simulink model "SOC_Estimation"  (R2019b)
settings: configuration reference "BMS_Sw_CodeGenConfig" (kept outside this file)
undefined symbols (not defined in the file): Battery, BMS_State_Enum, DiscIntNeverNeededParam, Ns_Module, NumModules, SOCInit, Ts
libraries: sharedTrackingLibrary x2, simulink x1
settings Model: DataDictionary=DD_SOC_Estimation.sldd  EnableAccessToBaseWorkspace=off  ExtModeTrigDuration=5  Creator=cpatel  LastModifiedBy=cpatel
settings ConfigSetRef: SourceName=BMS_Sw_CodeGenConfig

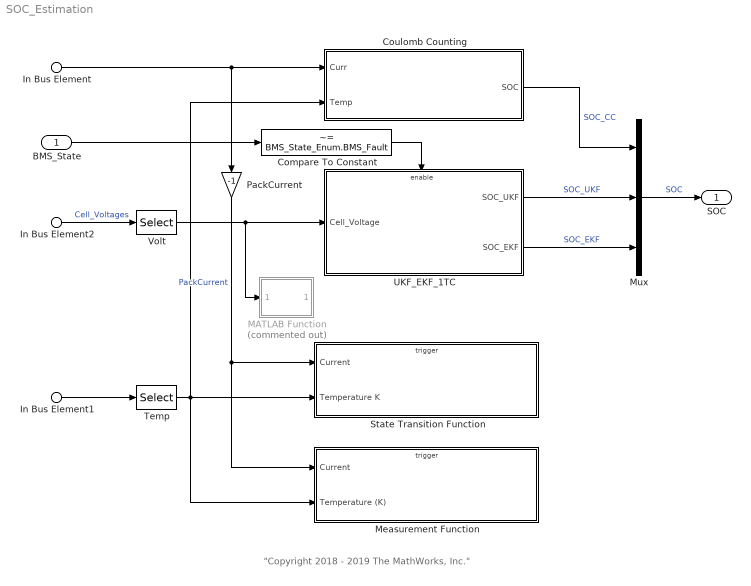
== system SOC_Estimation ==
  note: "Copyright 2018 - 2019 The MathWorks, Inc."
  BMS_State : Inport  OutDataTypeStr=Enum: BMS_State_Enum
  In Bus Element2 : Inport  Port=2  PortName=BMS_Input  Element=Cell_Voltages
  In Bus Element : Inport  Port=2  PortName=BMS_Input  Element=Pack_Current
  In Bus Element1 : Inport  Port=2  PortName=BMS_Input  Element=Cell_Temperatures
  Compare To Constant : simulink/Logic and Bit Operations/Compare To Constant  relop=~=  const=BMS_State_Enum.BMS_Fault  OutDataTypeStr=boolean
  Coulomb Counting : Subsystem  VariantControl=SocAlgo==1
  MATLAB Function : MATLAB Function  Commented=on  TreatAsAtomicUnit=on
  Measurement Function : Subsystem  TreatAsAtomicUnit=on
  Mux : Mux  Inputs=3
  PackCurrent : Gain  Gain=-1
  State Transition Function : Subsystem  TreatAsAtomicUnit=on
  Temp : Selector  InputPortWidth=Ns_Module*NumModules  IndexOptions=Index vector (dialog)  Indices=1  OutputSizes=1
  UKF_EKF_1TC : Subsystem  VariantControl=CellType==1
  Volt : Selector  InputPortWidth=Ns_Module*NumModules  IndexOptions=Index vector (dialog)  Indices=1  OutputSizes=1
  SOC : Outport  OutDataTypeStr=single  SampleTime=[0.10000000000000001,0]  VectorParamsAs1DForOutWhenUnconnected=off
  wires:
  In Bus Element2/1 -> Volt/1  "Cell_Voltages"
  In Bus Element1/1 -> Temp/1
  Mux/1 -> SOC/1  "SOC"
  Coulomb Counting/1(SOC) -> Mux/1  "SOC_CC"
  In Bus Element/1 -> PackCurrent/1, Coulomb Counting/1(Curr)
  UKF_EKF_1TC/1(SOC_UKF) -> Mux/2  "SOC_UKF"
  UKF_EKF_1TC/2(SOC_EKF) -> Mux/3  "SOC_EKF"
  BMS_State/1 -> Compare To Constant/1
  Compare To Constant/1 -> UKF_EKF_1TC/Enable
  PackCurrent/1 -> State Transition Function/1(Current), Measurement Function/1(Current)  "PackCurrent"
  Temp/1 -> State Transition Function/2(Temperature K), Measurement Function/2(Temperature (K)), Coulomb Counting/2(Temp)
  Volt/1 -> UKF_EKF_1TC/1(Cell_Voltage), MATLAB Function/1(meas)

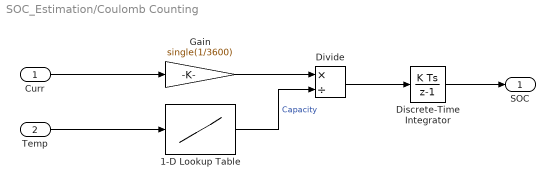
== system SOC_Estimation/Coulomb Counting ==
  Curr : Inport
  Temp : Inport  Port=2
  1-D Lookup Table : Lookup_n-D  NumberOfTableDimensions=1  BreakpointsForDimension1=single(Battery(1).Temperature_LUT)  Table=single(Battery(1).Capacity_LUT)  InternalRulePriority=Speed  RndMeth=Simplest  InputSameDT=on
  Discrete-Time Integrator : DiscreteIntegrator  InitialCondition=single(SOCInit+0.05)  SampleTime=-1  LimitOutput=on  UpperSaturationLimit=1  LowerSaturationLimit=0  ICPrevOutput=DiscIntNeverNeededParam  ICPrevScaledInput=DiscIntNeverNeededParam
  Divide : Product  Inputs=*/
  Gain : Gain  Gain=single(1/3600)
  SOC : Outport  VectorParamsAs1DForOutWhenUnconnected=off
  wires:
  Discrete-Time Integrator/1 -> SOC/1
  Curr/1 -> Gain/1
  Gain/1 -> Divide/1
  Divide/1 -> Discrete-Time Integrator/1
  1-D Lookup Table/1 -> Divide/2  "Capacity"
  Temp/1 -> 1-D Lookup Table/1

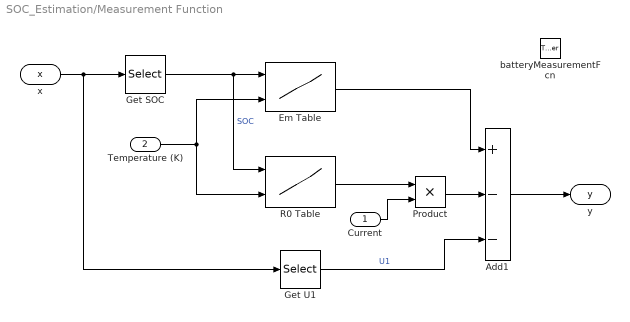
== system SOC_Estimation/Measurement Function ==
  Current : Inport
  Temperature (K) : Inport  Port=2
  batteryMeasurementFcn : TriggerPort  TriggerType=function-call  IsSimulinkFunction=on  FunctionName=batteryMeasurementFcn  VariantControl=Variant
  Add1 : Sum  Inputs=+--
  Em Table : Lookup_n-D  BreakpointsForDimension1=Battery.SOC_LUT  BreakpointsForDimension2=Battery.Temperature_LUT  BeginIndexSearchUsingPreviousIndexResult=on  Table=Battery.Em_LUT  ExtrapMethod=Clip  InternalRulePriority=Speed  RndMeth=Simplest  InputSameDT=on
  Get SOC : Selector  InputPortWidth=2  IndexOptions=Index vector (dialog)  Indices=[1]  OutputSizes=1
  Get U1 : Selector  InputPortWidth=2  IndexOptions=Index vector (dialog)  Indices=2  OutputSizes=1
  Product : Product
  R0 Table : Lookup_n-D  BreakpointsForDimension1=Battery.SOC_LUT  BreakpointsForDimension2=Battery.Temperature_LUT  BeginIndexSearchUsingPreviousIndexResult=on  Table=Battery.R0_LUT  ExtrapMethod=Clip  InternalRulePriority=Speed  RndMeth=Simplest  InputSameDT=on
  x : ArgIn  DisableCoverage=on  OutDataTypeStr=single  PortDimensions=2  ArgumentName=x
  y : ArgOut  DisableCoverage=on  OutDataTypeStr=single  ArgumentName=y
  wires:
  Get U1/1 -> Add1/3  "U1"
  Product/1 -> Add1/2
  Current/1 -> Product/2
  R0 Table/1 -> Product/1
  Temperature (K)/1 -> Em Table/2, R0 Table/2
  Add1/1 -> y/1
  Em Table/1 -> Add1/1
  Get SOC/1 -> Em Table/1, R0 Table/1  "SOC"
  x/1 -> Get SOC/1, Get U1/1

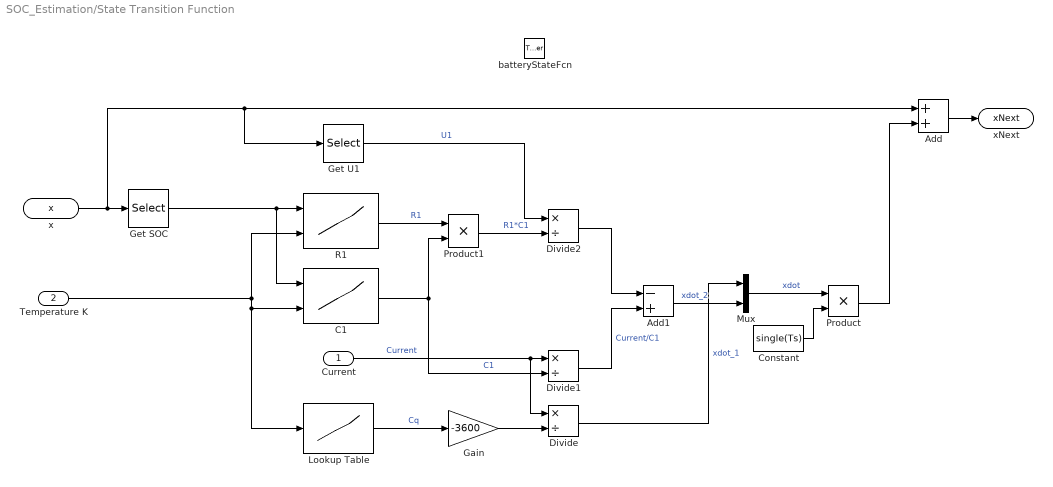
== system SOC_Estimation/State Transition Function ==
  Current : Inport
  Temperature K : Inport  Port=2
  batteryStateFcn : TriggerPort  TriggerType=function-call  IsSimulinkFunction=on  FunctionName=batteryStateFcn  VariantControl=Variant
  Add : Sum
  Add1 : Sum  Inputs=-+
  C1 : Lookup_n-D  BreakpointsForDimension1=Battery.SOC_LUT  BreakpointsForDimension2=Battery.Temperature_LUT  BeginIndexSearchUsingPreviousIndexResult=on  Table=Battery.C1_LUT  ExtrapMethod=Clip  InternalRulePriority=Speed  RndMeth=Simplest  InputSameDT=on
  Constant : Constant  Value=single(Ts)  OutDataTypeStr=single
  Divide : Product  Inputs=*/
  Divide1 : Product  Inputs=*/
  Divide2 : Product  Inputs=*/
  Gain : Gain  Gain=-3600
  Get SOC : Selector  InputPortWidth=2  IndexOptions=Index vector (dialog)  Indices=1  OutputSizes=1
  Get U1 : Selector  InputPortWidth=2  IndexOptions=Index vector (dialog)  Indices=2  OutputSizes=1
  Lookup Table : Lookup_n-D  NumberOfTableDimensions=1  BreakpointsForDimension1=Battery.Temperature_LUT  BeginIndexSearchUsingPreviousIndexResult=on  Table=Battery.Capacity_LUT  InternalRulePriority=Speed  RndMeth=Simplest  InputSameDT=on
  Mux : Mux  Inputs=2
  Product : Product  OutDataTypeStr=single
  Product1 : Product
  R1 : Lookup_n-D  BreakpointsForDimension1=Battery.SOC_LUT  BreakpointsForDimension2=Battery.Temperature_LUT  BeginIndexSearchUsingPreviousIndexResult=on  Table=Battery.R1_LUT  ExtrapMethod=Clip  InternalRulePriority=Speed  RndMeth=Simplest  InputSameDT=on
  x : ArgIn  DisableCoverage=on  OutDataTypeStr=single  PortDimensions=2  ArgumentName=x
  xNext : ArgOut  DisableCoverage=on  OutDataTypeStr=single  PortDimensions=2  ArgumentName=xNext
  wires:
  Lookup Table/1 -> Gain/1  "Cq"
  Product/1 -> Add/2
  Constant/1 -> Product/2
  Current/1 -> Divide1/1, Divide/1  "Current"
  Get SOC/1 -> C1/1, R1/1
  Temperature K/1 -> Lookup Table/1, C1/2, R1/2
  Add/1 -> xNext/1
  x/1 -> Add/1, Get U1/1, Get SOC/1
  Gain/1 -> Divide/2
  Divide/1 -> Mux/1  "xdot_1"
  Get U1/1 -> Divide2/1  "U1"
  Product1/1 -> Divide2/2  "R1*C1"
  R1/1 -> Product1/1  "R1"
  C1/1 -> Product1/2, Divide1/2  "C1"
  Divide1/1 -> Add1/2  "Current/C1"
  Divide2/1 -> Add1/1
  Add1/1 -> Mux/2  "xdot_2"
  Mux/1 -> Product/1  "xdot"

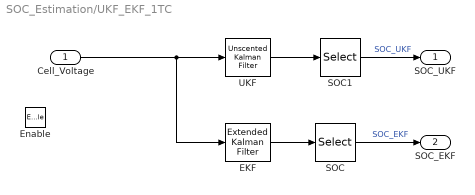
== system SOC_Estimation/UKF_EKF_1TC ==
  Cell_Voltage : Inport
  Enable : EnablePort
  EKF : sharedTrackingLibrary/Extended Kalman Filter  StateTransitionFcn=batteryStateFcn  HasStateTransitionJacobianFcn=off  HasAdditiveProcessNoise=Additive  ProcessNoise=1e-10*eye(2)  HasTimeVaryingProcessNoise=off  HasStateTransitionFcnExtraArgument=0  InitialState=[single(SOCInit+0.05); 0;]  InitialStateCovariance=[1e-5 1]  MeasurementFcn1=batteryMeasurementFcn  HasMeasurementJacobianFcn1=off  HasMeasurementEnablePort1=off  HasAdditiveMeasurementNoise1=Additive  MeasurementNoise1=1e-1  HasTimeVaryingMeasurementNoise1=off  HasMeasurementFcnExtraArgument1=0  MeasurementFcn2=myMeasurementFcn  HasMeasurementJacobianFcn2=off  HasMeasurementEnablePort2=off  HasAdditiveMeasurementNoise2=Additive  MeasurementNoise2=1  HasTimeVaryingMeasurementNoise2=off  HasMeasurementFcnExtraArgument2=0  MeasurementFcn3=myMeasurementFcn  HasMeasurementJacobianFcn3=off  HasMeasurementEnablePort3=off  HasAdditiveMeasurementNoise3=Additive  MeasurementNoise3=1  HasTimeVaryingMeasurementNoise3=off  HasMeasurementFcnExtraArgument3=0  MeasurementFcn4=myMeasurementFcn  HasMeasurementJacobianFcn4=off  HasMeasurementEnablePort4=off  HasAdditiveMeasurementNoise4=Additive  MeasurementNoise4=1  HasTimeVaryingMeasurementNoise4=off  HasMeasurementFcnExtraArgument4=0  MeasurementFcn5=myMeasurementFcn  HasMeasurementJacobianFcn5=off  HasMeasurementEnablePort5=off  HasAdditiveMeasurementNoise5=Additive  MeasurementNoise5=1  HasTimeVaryingMeasurementNoise5=off  HasMeasurementFcnExtraArgument5=0  EnableMultirate=off  StateTransitionFcnSampleTime=1  MeasurementFcn1SampleTime=1  MeasurementFcn2SampleTime=1  MeasurementFcn3SampleTime=1  MeasurementFcn4SampleTime=1  MeasurementFcn5SampleTime=1  UseCurrentEstimator=on  OutputStateCovariance=off  DataType=single  SampleTime=Ts  NumberOfMeasurements=1
      settings: SourceProductName=Control System Toolbox  SourceProductBaseCode=CT
  SOC : Selector  InputPortWidth=2  IndexOptions=Index vector (dialog)  Indices=1  OutputSizes=1
  SOC1 : Selector  InputPortWidth=2  IndexOptions=Index vector (dialog)  Indices=1  OutputSizes=1
  UKF : sharedTrackingLibrary/Unscented Kalman Filter  StateTransitionFcn=batteryStateFcn  HasAdditiveProcessNoise=Additive  ProcessNoise=1e-10*eye(2)  HasTimeVaryingProcessNoise=off  HasStateTransitionFcnExtraArgument=0  InitialState=[single(SOCInit+0.05); 0;]  InitialStateCovariance=[1e-5 1]  Alpha=1  Beta=2  Kappa=1  MeasurementFcn1=batteryMeasurementFcn  HasMeasurementEnablePort1=off  HasAdditiveMeasurementNoise1=Additive  MeasurementNoise1=0.1  HasTimeVaryingMeasurementNoise1=off  HasMeasurementFcnExtraArgument1=0  MeasurementFcn2=myMeasurementFcn  HasMeasurementEnablePort2=off  HasAdditiveMeasurementNoise2=Additive  MeasurementNoise2=1  HasTimeVaryingMeasurementNoise2=off  HasMeasurementFcnExtraArgument2=0  MeasurementFcn3=myMeasurementFcn  HasMeasurementEnablePort3=off  HasAdditiveMeasurementNoise3=Additive  MeasurementNoise3=1  HasTimeVaryingMeasurementNoise3=off  HasMeasurementFcnExtraArgument3=0  MeasurementFcn4=myMeasurementFcn  HasMeasurementEnablePort4=off  HasAdditiveMeasurementNoise4=Additive  MeasurementNoise4=1  HasTimeVaryingMeasurementNoise4=off  HasMeasurementFcnExtraArgument4=0  MeasurementFcn5=myMeasurementFcn  HasMeasurementEnablePort5=off  HasAdditiveMeasurementNoise5=Additive  MeasurementNoise5=1  HasTimeVaryingMeasurementNoise5=off  HasMeasurementFcnExtraArgument5=0  EnableMultirate=off  StateTransitionFcnSampleTime=-1  MeasurementFcn1SampleTime=-1  MeasurementFcn2SampleTime=-1  MeasurementFcn3SampleTime=-1  MeasurementFcn4SampleTime=-1  MeasurementFcn5SampleTime=-1  UseCurrentEstimator=on  OutputStateCovariance=off  DataType=single  SampleTime=Ts  NumberOfMeasurements=1
      settings: SourceProductName=Control System Toolbox  SourceProductBaseCode=CT
  SOC_UKF : Outport  VectorParamsAs1DForOutWhenUnconnected=off
  SOC_EKF : Outport  Port=2  VectorParamsAs1DForOutWhenUnconnected=off
  wires:
  UKF/1 -> SOC1/1
  Cell_Voltage/1 -> UKF/1, EKF/1
  SOC1/1 -> SOC_UKF/1  "SOC_UKF"
  EKF/1 -> SOC/1
  SOC/1 -> SOC_EKF/1  "SOC_EKF"

== matlab function SOC_Estimation/MATLAB Function ==
  data: meas input double; xhatOut output double
function xhatOut  = EXTKALMAN(meas)
%EXTKALMAN Radar Data Processing Tracker Using an Extended Kalman Filter
%
%  This program is executed as a MATLAB function block in the 
%  sldemo_radar Simulink model.  The estimated and actual positions are 
%  saved to the workspace and are plotted at the end of the simulation by 
%  the program aero_radplot (called from the simulation automatically).
%
%

%  Copyright 1990-2013 The MathWorks, Inc.
deltat = 0.1;
% Initialization
persistent P;
persistent xhat
if isempty(P)
    xhat = [0.75; 0];
    P = 1e-10*eye(2);
end
    
%  Radar update time deltat is inherited from model workspace

% 1. Compute Phi, Q, and R 
Phi = [1 deltat; 0 1];
%Phi = deltat;
Q =  1e-10*eye(2);
R =  1e-1;

% 2. Propagate the covariance matrix:
P = Phi*P*Phi' + Q;

% 3. Propagate the track estimate::
xhat = Phi*xhat;

% 4 a). Compute observation estimates:
xNext = batteryStateFnc(xhat);

% 4 b). Compute observation vector y and linearized measurement matrix M 
yhat = batteryMeasurementFcn(xhat);
M = [ cos(xNext(1))          0 sin(xNext(1))          0
   -sin(xNext(1))/xNext(2) 0 cos(xNext(1))/xNext(2) 0 ];
% 4 c).  Compute residual (Estimation Error)
residual = meas - yhat;

% 5. Compute Kalman Gain:
W = P*M'*inv(M*P*M'+ R);

% 6. Update estimate
xhat = xhat + W*residual;

% 7. Update Covariance Matrix
P = (eye(4)-W*M)*P*(eye(4)-W*M)' + W*R*W';

xhatOut = xhat;
